simulink model "model1"  (R2022a)
settings: Solver=VariableStepAuto  StartTime=0.0  StopTime=2.99  RelTol=1e-3
undefined symbols (not defined in the file): A, B, C, D, K, x_0
settings Model: Creator=Family  LastModifiedBy=Family

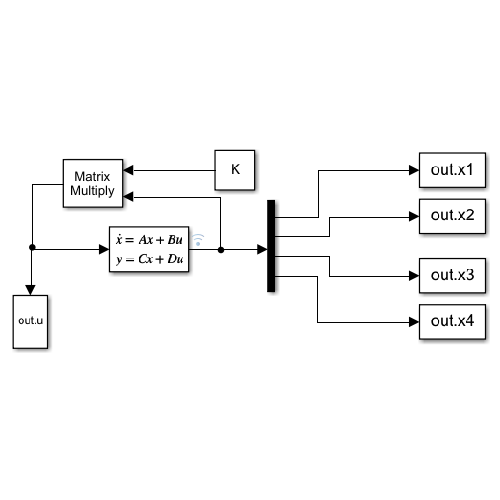
[thumbnail: Simulink's stored preview of the top-level diagram]
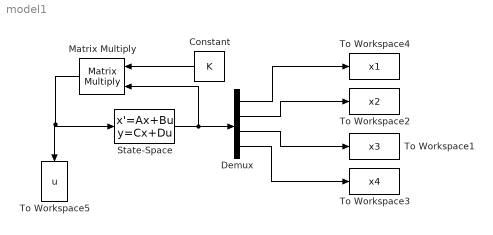
== system model1 ==
  Constant : Constant  Value=K  VectorParams1D=off
  Demux : Demux
  Matrix Multiply : Product  Multiplication=Matrix(*)
  State-Space : StateSpace  A=A  B=B  C=C  D=D  InitialCondition=x_0  ParameterTunability=Unconstrained
  To Workspace1 : ToWorkspace  VariableName=x3  SaveFormat=Timeseries  SampleTime=-1
  To Workspace2 : ToWorkspace  VariableName=x2  SaveFormat=Timeseries  SampleTime=-1
  To Workspace3 : ToWorkspace  VariableName=x4  SaveFormat=Timeseries  SampleTime=-1
  To Workspace4 : ToWorkspace  VariableName=x1  SaveFormat=Timeseries  SampleTime=0.00001
  To Workspace5 : ToWorkspace  VariableName=u  SaveFormat=Timeseries  SampleTime=-1
  wires:
  Matrix Multiply/1 -> State-Space/1, To Workspace5/1
  Constant/1 -> Matrix Multiply/1
  Demux/1 -> To Workspace4/1
  State-Space/1 -> Matrix Multiply/2, Demux/1
  Demux/4 -> To Workspace3/1
  Demux/2 -> To Workspace2/1
  Demux/3 -> To Workspace1/1
